simulink model "LQR_test"  (R2023b)
settings: Solver=VariableStepAuto  StartTime=0.0  StopTime=10.0  RelTol=1e-3
values from neighbouring files (symbols this model uses):
  A_d = eye(size(Ac)) + Ts * Ac    [closed_loop_identification.m]
  B_d = Ts * Bc    [closed_loop_identification.m]
  C_d = Cc    [closed_loop_identification.m]
  D_d = Dc    [closed_loop_identification.m]
  K = dlqr(A_d, B_d, Q, R)    [LQR_tuning.m]    (also in LQR_tuning_continous.m = lqr(ss_continous.A, ss_continous.B, Q, R); LQR_tuning_discrete.m = dlqr(ss_object_discrete.A, ss_object_discrete.B, Q, R))
  tf_object_discrete = tf(ss_object_discrete)    [closed_loop_identification.m]
  Ts = 0.002    [closed_loop_identification.m]    (also in closed_loop_identification_LS.m = 0.001; init.m = 0.001)
undefined symbols (not defined in the file or in its folder): Discrete, Time
libraries: ctrlSharedLib x1
settings Model: Creator=User  LastModifiedBy=User

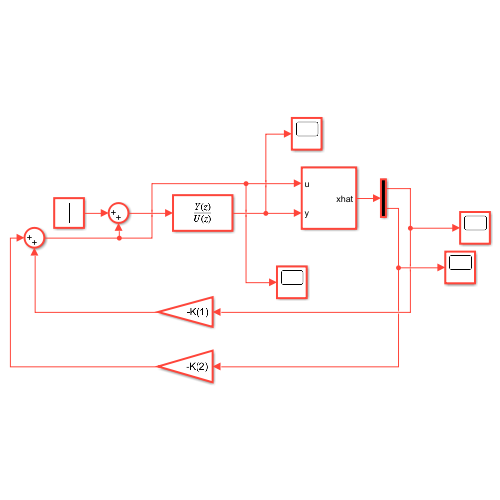
[thumbnail: Simulink's stored preview of the top-level diagram]
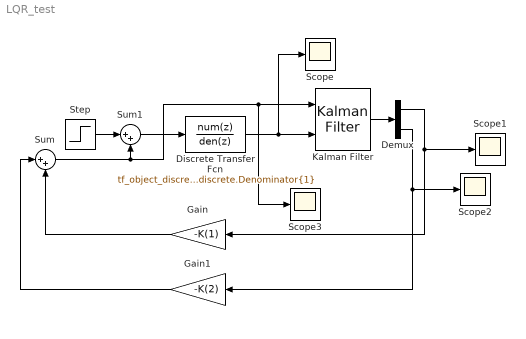
== system LQR_test ==
  Demux : Demux  Outputs=2
  Discrete Transfer Fcn : DiscreteTransferFcn  Numerator=tf_object_discrete.Numerator{1}  Denominator=tf_object_discrete.Denominator{1}
  Gain : Gain  Gain=-K(1)
  Gain1 : Gain  Gain=-K(2)
  Kalman Filter : ctrlSharedLib/Kalman Filter  TimeDomain=Discrete-Time  UseCurrentEstimator=on  ModelSource=Individual A, B, C, D matrices  ModelSourceVariable=ss(0.95,1,1,0,1)  A=A_d  B=B_d  C=C_d  D=D_d  NumberOfStates=1  NumberOfInputs=1  NumberOfOutputs=1  InitialEstimateSource=Dialog  X0=0  P0=10  UseK=off  UseGH=off  NumberOfProcessNoiseInputs=1  G=1  TimeInvariantG=on  H=0  TimeInvariantH=on  Q=0.05  TimeInvariantQ=on  R=1  TimeInvariantR=on  N=0  TimeInvariantN=on  AddInputPort=on  AddEnablePort=off  OutputEstimatedY=off  OutputP=off  Ts=-1
  Scope{,1..3} (4 alike) : Scope
  Step : Step  After=0.1  SampleTime=Ts
  Sum : Sum  Inputs=|++
  Sum1 : Sum  Inputs=|++
  wires:
  Discrete Transfer Fcn/1 -> Scope/1, Kalman Filter/2
  Gain/1 -> Sum/2
  Gain1/1 -> Sum/1
  Step/1 -> Sum1/1
  Sum/1 -> Scope3/1, Kalman Filter/1, Sum1/2
  Sum1/1 -> Discrete Transfer Fcn/1
  Kalman Filter/1 -> Demux/1
  Demux/1 -> Scope1/1, Gain/1
  Demux/2 -> Scope2/1, Gain1/1
